simulink model "proj_pid"  (R2021a)
settings: Solver=VariableStepAuto  StartTime=0.0  StopTime=1000  RelTol=1e-3
values from neighbouring files (symbols this model uses):
  A = [0 0 1 0 ... (first row only)    [proj_LQRcode.m]    (also in proj_PIDcode.m)
  B = [0 0 ... (first row only)    [proj_LQRcode.m]    (also in proj_PIDcode.m)
  C = [1 0 0 0 ... (first row only)    [proj_LQRcode.m]    (also in proj_PIDcode.m)
  initialstate = [-3.1;-39.16;0.00002;0.0041]    [proj_PIDcode.m]
  kd1 = 500    [proj_PIDcode.m]
  kd2 = 150.643    [proj_PIDcode.m]
  ki1 = 1.7    [proj_PIDcode.m]
  ki2 = 0.005    [proj_PIDcode.m]
  kp1 = 4.5    [proj_PIDcode.m]
  kp2 = 1.35    [proj_PIDcode.m]
settings Model: Creator=huangzijing  LastModifiedBy=huangzijing

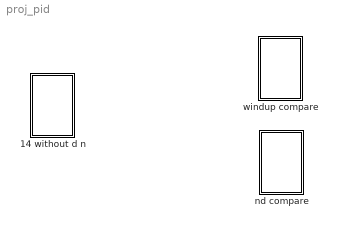
== system proj_pid ==
  14 without d n : Subsystem
  nd compare : Subsystem
  windup compare : Subsystem

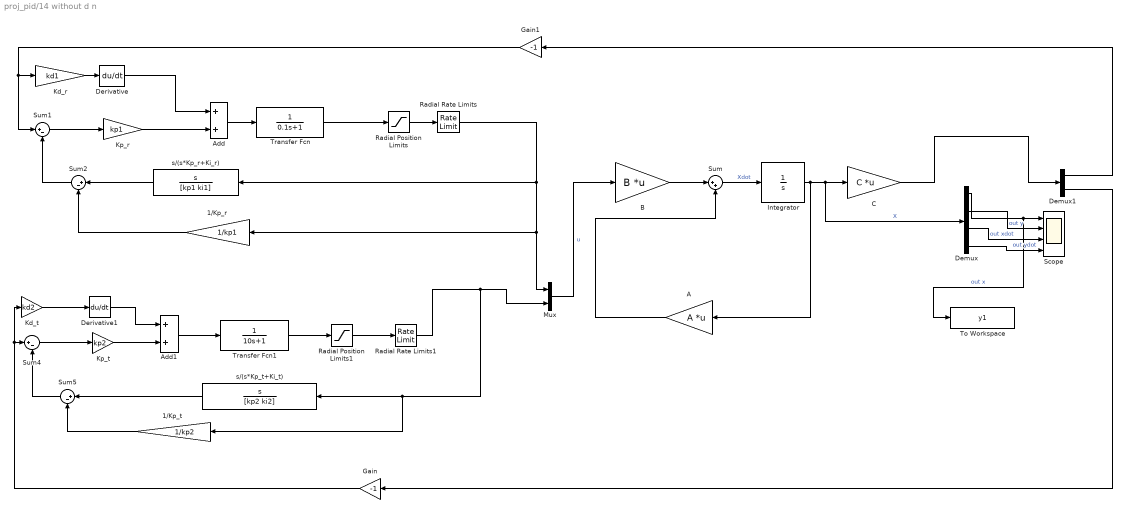
== system proj_pid/14 without d n ==
  1/Kp_r : Gain  Gain=1/kp1
  1/Kp_t : Gain  Gain=1/kp2
  A : Gain  Gain=A  Multiplication=Matrix(K*u)
  Add : Sum
  Add1 : Sum
  B : Gain  Gain=B  Multiplication=Matrix(K*u)
  C : Gain  Gain=C  Multiplication=Matrix(K*u)
  Demux : Demux
  Demux1 : Demux  Outputs=2
  Derivative : Derivative
  Derivative1 : Derivative
  Gain : Gain  Gain=-1
  Gain1 : Gain  Gain=-1
  Integrator : Integrator  InitialCondition=initialstate
  Kd_r : Gain  Gain=kd1
  Kd_t : Gain  Gain=kd2
  Kp_r : Gain  Gain=kp1
  Kp_t : Gain  Gain=kp2
  Mux : Mux  Inputs=2
  Radial Position Limits : Saturate  UpperLimit=5880  LowerLimit=-5880
  Radial Position Limits1 : Saturate  UpperLimit=820  LowerLimit=-820
  Radial Rate Limits : RateLimiter  RisingSlewLimit=30  FallingSlewLimit=-30  SampleTimeMode=inherited
  Radial Rate Limits1 : RateLimiter  RisingSlewLimit=500  FallingSlewLimit=-500  SampleTimeMode=inherited
  Scope : Scope  NumInputPorts=4
  Sum : Sum  Inputs=|++
  Sum{1..2,4..5} (4 alike) : Sum  Inputs=|+-
  To Workspace : ToWorkspace  VariableName=y1  SaveFormat=Timeseries  SampleTime=-1
  Transfer Fcn : TransferFcn  Denominator=[0.1 1]
  Transfer Fcn1 : TransferFcn  Denominator=[10 1]
  s/(s*Kp_r+Ki_r) : TransferFcn  Numerator=[1 0]  Denominator=[kp1 ki1]
  s/(s*Kp_t+Ki_t) : TransferFcn  Numerator=[1 0]  Denominator=[kp2 ki2]
  wires:
  Demux/3 -> Scope/3  "out xdot"
  Radial Position Limits1/1 -> Radial Rate Limits1/1
  Mux/1 -> B/1  "u"
  Sum/1 -> Integrator/1  "Xdot"
  Transfer Fcn1/1 -> Radial Position Limits1/1
  Add/1 -> Transfer Fcn/1
  A/1 -> Sum/2
  Derivative1/1 -> Add1/1
  s/(s*Kp_t+Ki_t)/1 -> Sum5/1
  s/(s*Kp_r+Ki_r)/1 -> Sum2/1
  1/Kp_r/1 -> Sum2/2
  Demux1/1 -> Gain1/1
  Gain/1 -> Kd_t/1, Sum4/1
  Sum2/1 -> Sum1/2
  Demux/4 -> Scope/4  "out ydot"
  Kd_t/1 -> Derivative1/1
  Add1/1 -> Transfer Fcn1/1
  Kp_t/1 -> Add1/2
  Sum1/1 -> Kp_r/1
  Sum5/1 -> Sum4/2
  B/1 -> Sum/1
  Derivative/1 -> Add/1
  Kd_r/1 -> Derivative/1
  Demux/2 -> Scope/2  "out y"
  Demux/1 -> To Workspace/1, Scope/1  "out x"
  C/1 -> Demux1/1
  Kp_r/1 -> Add/2
  Radial Position Limits/1 -> Radial Rate Limits/1
  Radial Rate Limits1/1 -> 1/Kp_t/1, s/(s*Kp_t+Ki_t)/1, Mux/2
  Integrator/1 -> Demux/1, C/1, A/1  "X"
  Gain1/1 -> Sum1/1, Kd_r/1
  Radial Rate Limits/1 -> 1/Kp_r/1, Mux/1, s/(s*Kp_r+Ki_r)/1
  Demux1/2 -> Gain/1
  1/Kp_t/1 -> Sum5/2
  Sum4/1 -> Kp_t/1
  Transfer Fcn/1 -> Radial Position Limits/1

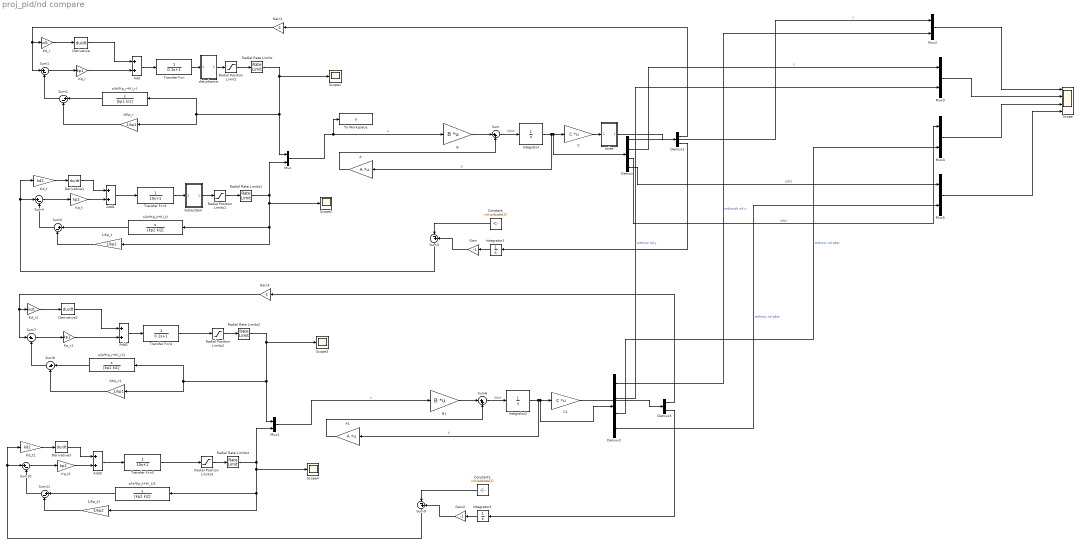
== system proj_pid/nd compare ==
  1/Kp_r : Gain  Gain=1/kp1
  1/Kp_r1 : Gain  Gain=1/kp1
  1/Kp_t : Gain  Gain=1/kp2
  1/Kp_t1 : Gain  Gain=1/kp2
  A : Gain  Gain=A  Multiplication=Matrix(K*u)
  A1 : Gain  Gain=A  Multiplication=Matrix(K*u)
  Add{,1..3} (4 alike) : Sum
  B : Gain  Gain=B  Multiplication=Matrix(K*u)
  B1 : Gain  Gain=B  Multiplication=Matrix(K*u)
  C : Gain  Gain=C  Multiplication=Matrix(K*u)
  C1 : Gain  Gain=C  Multiplication=Matrix(K*u)
  Constant : Constant  Value=initialstate(2)
  Constant1 : Constant  Value=initialstate(2)
  Demux : Demux
  Demux1 : Demux  Outputs=2
  Demux2 : Demux
  Demux3 : Demux  Outputs=2
  Derivative{,1..3} (4 alike) : Derivative
  Gain{,1..3} (4 alike) : Gain  Gain=-1
  Integrator : Integrator  InitialCondition=initialstate
  Integrator1 : Integrator
  Integrator2 : Integrator  InitialCondition=initialstate
  Integrator3 : Integrator
  Kd_r : Gain  Gain=kd1
  Kd_r1 : Gain  Gain=kd1
  Kd_t : Gain  Gain=kd2
  Kd_t1 : Gain  Gain=kd2
  Kp_r : Gain  Gain=kp1
  Kp_r1 : Gain  Gain=kp1
  Kp_t : Gain  Gain=kp2
  Kp_t1 : Gain  Gain=kp2
  Mux{,1..5} (6 alike) : Mux  Inputs=2
  Radial Position Limits : Saturate  UpperLimit=5880  LowerLimit=-5880
  Radial Position Limits1 : Saturate  UpperLimit=820  LowerLimit=-820
  Radial Position Limits2 : Saturate  UpperLimit=5880  LowerLimit=-5880
  Radial Position Limits3 : Saturate  UpperLimit=820  LowerLimit=-820
  Radial Rate Limits : RateLimiter  RisingSlewLimit=30  FallingSlewLimit=-30  SampleTimeMode=inherited
  Radial Rate Limits1 : RateLimiter  RisingSlewLimit=500  FallingSlewLimit=-500  SampleTimeMode=inherited
  Radial Rate Limits2 : RateLimiter  RisingSlewLimit=30  FallingSlewLimit=-30  SampleTimeMode=inherited
  Radial Rate Limits3 : RateLimiter  RisingSlewLimit=500  FallingSlewLimit=-500  SampleTimeMode=inherited
  Scope : Scope  NumInputPorts=4
  Scope{1..4} (4 alike) : Scope
  Subsystem : Subsystem
  Sum : Sum  Inputs=|++
  Sum{1..2,4..5,7..8,10..11} (8 alike) : Sum  Inputs=|+-
  Sum3 : Sum  Inputs=|-+
  Sum6 : Sum  Inputs=|++
  Sum9 : Sum  Inputs=|-+
  To Workspace : ToWorkspace  VariableName=u  SampleTime=-1
      settings: Save2DSignal=2-D array (concatenate along first dimension)
  Transfer Fcn : TransferFcn  Denominator=[0.1 1]
  Transfer Fcn1 : TransferFcn  Denominator=[10 1]
  Transfer Fcn2 : TransferFcn  Denominator=[0.1 1]
  Transfer Fcn3 : TransferFcn  Denominator=[10 1]
  disturbance : Subsystem
  "noise " : Subsystem
  s/(s*Kp_r+Ki_r) : TransferFcn  Numerator=[1 0]  Denominator=[kp1 ki1]
  s/(s*Kp_r+Ki_r)1 : TransferFcn  Numerator=[1 0]  Denominator=[kp1 ki1]
  s/(s*Kp_t+Ki_t) : TransferFcn  Numerator=[1 0]  Denominator=[kp2 ki2]
  s/(s*Kp_t+Ki_t)1 : TransferFcn  Numerator=[1 0]  Denominator=[kp2 ki2]
  wires:
  Sum6/1 -> Integrator2/1  "Xdot"
  Integrator3/1 -> Gain2/1
  Demux2/4 -> Mux5/2  "without nd ydot"
  Sum2/1 -> Sum1/2
  Demux1/1 -> Gain1/1
  Sum11/1 -> Sum10/2
  B1/1 -> Sum6/1
  Demux3/1 -> Gain3/1
  Radial Position Limits2/1 -> Radial Rate Limits2/1
  Sum4/1 -> Kp_t/1
  Transfer Fcn2/1 -> Radial Position Limits2/1
  Mux/1 -> To Workspace/1, B/1  "u"
  Add/1 -> Transfer Fcn/1
  Demux2/1 -> Mux2/2  "withouth nd x"
  s/(s*Kp_t+Ki_t)1/1 -> Sum11/1
  Integrator/1 -> Demux/1, C/1, A/1  "X"
  Transfer Fcn3/1 -> Radial Position Limits3/1
  Constant/1 -> Sum3/1
  Transfer Fcn1/1 -> Subsystem/1(In1)
  Kd_r1/1 -> Derivative2/1
  Radial Position Limits/1 -> Radial Rate Limits/1
  Derivative3/1 -> Add3/1
  Mux3/1 -> Scope/2
  Transfer Fcn/1 -> disturbance/1(In1)
  Add3/1 -> Transfer Fcn3/1
  Mux1/1 -> B1/1  "u"
  Demux2/3 -> Mux4/2  "without nd xdot"
  s/(s*Kp_r+Ki_r)1/1 -> Sum8/1
  Sum10/1 -> Kp_t1/1
  1/Kp_t/1 -> Sum5/2
  Sum1/1 -> Kp_r/1
  1/Kp_r1/1 -> Sum8/2
  Kp_t1/1 -> Add3/2
  Mux4/1 -> Scope/3
  s/(s*Kp_r+Ki_r)/1 -> Sum2/1
  Gain1/1 -> Sum1/1, Kd_r/1
  Demux/4 -> Mux5/1  "ydot"
  Gain2/1 -> Sum9/2
  Kp_t/1 -> Add1/2
  Derivative1/1 -> Add1/1
  1/Kp_t1/1 -> Sum11/2
  Sum/1 -> Integrator/1  "Xdot"
  Sum8/1 -> Sum7/2
  Sum3/1 -> Kd_t/1, Sum4/1
  Gain3/1 -> Sum7/1, Kd_r1/1
  Sum5/1 -> Sum4/2
  Constant1/1 -> Sum9/1
  1/Kp_r/1 -> Sum2/2
  Radial Position Limits3/1 -> Radial Rate Limits3/1
  Mux5/1 -> Scope/4
  Radial Rate Limits3/1 -> Scope4/1, s/(s*Kp_t+Ki_t)1/1, 1/Kp_t1/1, Mux1/2
  Sum9/1 -> Kd_t1/1, Sum10/1
  B/1 -> Sum/1
  Kp_r/1 -> Add/2
  Derivative/1 -> Add/1
  Demux/3 -> Mux4/1  "xdot"
  Subsystem/1(Out1) -> Radial Position Limits1/1
  C/1 -> "noise "/1(In1)
  Radial Rate Limits1/1 -> Scope2/1, s/(s*Kp_t+Ki_t)/1, 1/Kp_t/1, Mux/2
  "noise "/1(Out1) -> Demux1/1
  Demux/2 -> Mux3/1  "y"
  A/1 -> Sum/2
  Kd_t1/1 -> Derivative3/1
  Demux/1 -> Mux2/1  "x"
  Demux1/2 -> Integrator1/1
  Radial Rate Limits2/1 -> Scope3/1, s/(s*Kp_r+Ki_r)1/1, 1/Kp_r1/1, Mux1/1
  Mux2/1 -> Scope/1
  Add2/1 -> Transfer Fcn2/1
  Gain/1 -> Sum3/2
  Add1/1 -> Transfer Fcn1/1
  s/(s*Kp_t+Ki_t)/1 -> Sum5/1
  Kd_r/1 -> Derivative/1
  Demux2/2 -> Mux3/2  "without nd y"
  C1/1 -> Demux3/1
  Derivative2/1 -> Add2/1
  Radial Position Limits1/1 -> Radial Rate Limits1/1
  Kd_t/1 -> Derivative1/1
  Radial Rate Limits/1 -> Scope1/1, s/(s*Kp_r+Ki_r)/1, 1/Kp_r/1, Mux/1
  Integrator2/1 -> Demux2/1, C1/1, A1/1  "X"
  Demux3/2 -> Integrator3/1
  Kp_r1/1 -> Add2/2
  Sum7/1 -> Kp_r1/1
  disturbance/1(Out1) -> Radial Position Limits/1
  A1/1 -> Sum6/2
  Integrator1/1 -> Gain/1

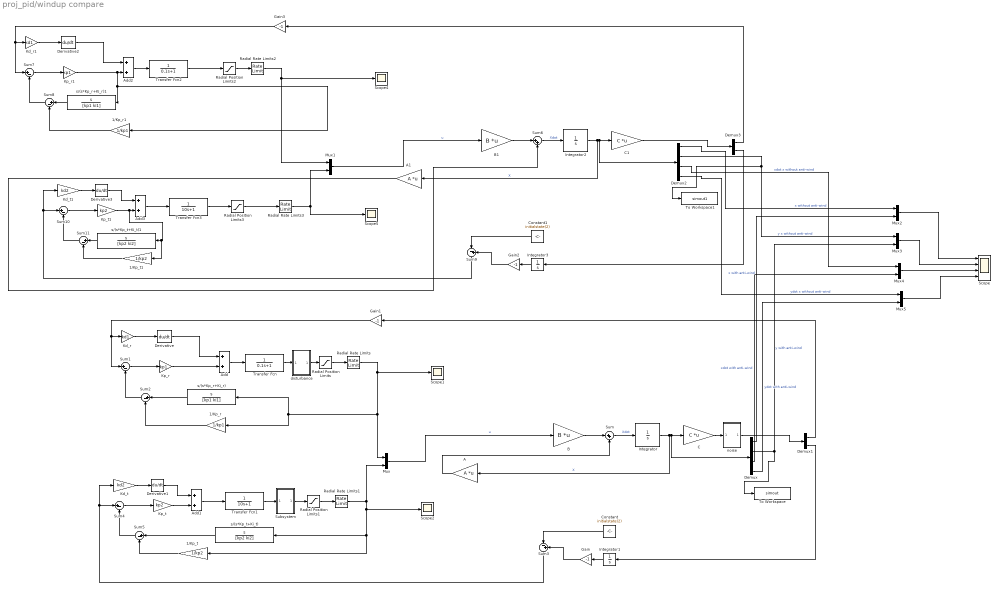
== system proj_pid/windup compare ==
  1/Kp_r : Gain  Gain=1/kp1
  1/Kp_r1 : Gain  Gain=1/kp1
  1/Kp_t : Gain  Gain=1/kp2
  1/Kp_t1 : Gain  Gain=1/kp2
  A : Gain  Gain=A  Multiplication=Matrix(K*u)
  A1 : Gain  Gain=A  Multiplication=Matrix(K*u)
  Add{,1..3} (4 alike) : Sum
  B : Gain  Gain=B  Multiplication=Matrix(K*u)
  B1 : Gain  Gain=B  Multiplication=Matrix(K*u)
  C : Gain  Gain=C  Multiplication=Matrix(K*u)
  C1 : Gain  Gain=C  Multiplication=Matrix(K*u)
  Constant : Constant  Value=initialstate(2)
  Constant1 : Constant  Value=initialstate(2)
  Demux : Demux
  Demux1 : Demux  Outputs=2
  Demux2 : Demux
  Demux3 : Demux  Outputs=2
  Derivative{,1..3} (4 alike) : Derivative
  Gain{,1..3} (4 alike) : Gain  Gain=-1
  Integrator : Integrator  InitialCondition=initialstate
  Integrator1 : Integrator
  Integrator2 : Integrator  InitialCondition=initialstate
  Integrator3 : Integrator
  Kd_r : Gain  Gain=kd1
  Kd_r1 : Gain  Gain=kd1
  Kd_t : Gain  Gain=kd2
  Kd_t1 : Gain  Gain=kd2
  Kp_r : Gain  Gain=kp1
  Kp_r1 : Gain  Gain=kp1
  Kp_t : Gain  Gain=kp2
  Kp_t1 : Gain  Gain=kp2
  Mux{,1..5} (6 alike) : Mux  Inputs=2
  Radial Position Limits : Saturate  UpperLimit=5880  LowerLimit=-5880
  Radial Position Limits1 : Saturate  UpperLimit=820  LowerLimit=-820
  Radial Position Limits2 : Saturate  UpperLimit=5880  LowerLimit=-5880
  Radial Position Limits3 : Saturate  UpperLimit=820  LowerLimit=-820
  Radial Rate Limits : RateLimiter  RisingSlewLimit=30  FallingSlewLimit=-30  SampleTimeMode=inherited
  Radial Rate Limits1 : RateLimiter  RisingSlewLimit=500  FallingSlewLimit=-500  SampleTimeMode=inherited
  Radial Rate Limits2 : RateLimiter  RisingSlewLimit=30  FallingSlewLimit=-30  SampleTimeMode=inherited
  Radial Rate Limits3 : RateLimiter  RisingSlewLimit=500  FallingSlewLimit=-500  SampleTimeMode=inherited
  Scope : Scope  NumInputPorts=4
  Scope{1..2,4..5} (4 alike) : Scope
  Subsystem : Subsystem
  Sum : Sum  Inputs=|++
  Sum{1..2,4..5,7..8,10..11} (8 alike) : Sum  Inputs=|+-
  Sum3 : Sum  Inputs=|-+
  Sum6 : Sum  Inputs=|++
  Sum9 : Sum  Inputs=|-+
  To Workspace : ToWorkspace  VariableName=simout  SaveFormat=Timeseries  SampleTime=-1
  To Workspace1 : ToWorkspace  VariableName=simout1  SaveFormat=Timeseries  SampleTime=-1
  Transfer Fcn : TransferFcn  Denominator=[0.1 1]
  Transfer Fcn1 : TransferFcn  Denominator=[10 1]
  Transfer Fcn2 : TransferFcn  Denominator=[0.1 1]
  Transfer Fcn3 : TransferFcn  Denominator=[10 1]
  disturbance : Subsystem
  "noise " : Subsystem
  s/(s*Kp_r+Ki_r) : TransferFcn  Numerator=[1 0]  Denominator=[kp1 ki1]
  s/(s*Kp_r+Ki_r)1 : TransferFcn  Numerator=[1 0]  Denominator=[kp1 ki1]
  s/(s*Kp_t+Ki_t) : TransferFcn  Numerator=[1 0]  Denominator=[kp2 ki2]
  s/(s*Kp_t+Ki_t)1 : TransferFcn  Numerator=[1 0]  Denominator=[kp2 ki2]
  wires:
  Sum/1 -> Integrator/1  "Xdot"
  B/1 -> Sum/1
  Integrator/1 -> Demux/1, C/1, A/1  "X"
  A/1 -> Sum/2
  Radial Rate Limits/1 -> Scope1/1, s/(s*Kp_r+Ki_r)/1, 1/Kp_r/1, Mux/1
  1/Kp_r/1 -> Sum2/2
  Kp_t/1 -> Add1/2
  Radial Position Limits/1 -> Radial Rate Limits/1
  Radial Position Limits1/1 -> Radial Rate Limits1/1
  Sum5/1 -> Sum4/2
  Radial Rate Limits1/1 -> Scope2/1, s/(s*Kp_t+Ki_t)/1, 1/Kp_t/1, Mux/2
  Sum2/1 -> Sum1/2
  1/Kp_t/1 -> Sum5/2
  Add/1 -> Transfer Fcn/1
  s/(s*Kp_r+Ki_r)/1 -> Sum2/1
  Kp_r/1 -> Add/2
  Derivative1/1 -> Add1/1
  Sum4/1 -> Kp_t/1
  Sum1/1 -> Kp_r/1
  Kd_t/1 -> Derivative1/1
  Kd_r/1 -> Derivative/1
  Add1/1 -> Transfer Fcn1/1
  s/(s*Kp_t+Ki_t)/1 -> Sum5/1
  Derivative/1 -> Add/1
  Mux/1 -> B/1  "u"
  Sum3/1 -> Kd_t/1, Sum4/1
  Demux1/2 -> Integrator1/1
  Constant/1 -> Sum3/1
  Integrator1/1 -> Gain/1
  Gain/1 -> Sum3/2
  Demux/2 -> Mux3/2, To Workspace/1  "y with anti-wind"
  Demux1/1 -> Gain1/1
  Gain1/1 -> Sum1/1, Kd_r/1
  Integrator3/1 -> Gain2/1
  Sum7/1 -> Kp_r1/1
  Kd_r1/1 -> Derivative2/1
  Integrator2/1 -> Demux2/1, C1/1, A1/1  "X"
  B1/1 -> Sum6/1
  Gain2/1 -> Sum9/2
  Sum6/1 -> Integrator2/1  "Xdot"
  Sum10/1 -> Kp_t1/1
  Radial Rate Limits2/1 -> Scope4/1, Mux1/1
  Radial Position Limits2/1 -> Radial Rate Limits2/1
  Mux1/1 -> B1/1  "u"
  Kp_t1/1 -> 1/Kp_t1/1, s/(s*Kp_t+Ki_t)1/1, Add3/2
  1/Kp_r1/1 -> Sum8/2
  Sum11/1 -> Sum10/2
  Radial Position Limits3/1 -> Radial Rate Limits3/1
  Radial Rate Limits3/1 -> Scope5/1, Mux1/2
  Sum8/1 -> Sum7/2
  Demux3/2 -> Integrator3/1
  1/Kp_t1/1 -> Sum11/2
  Demux2/1 -> Mux2/1  "x without anti-wind"
  Derivative3/1 -> Add3/1
  C1/1 -> Demux3/1
  Transfer Fcn3/1 -> Radial Position Limits3/1
  Kd_t1/1 -> Derivative3/1
  Add3/1 -> Transfer Fcn3/1
  s/(s*Kp_t+Ki_t)1/1 -> Sum11/1
  Transfer Fcn2/1 -> Radial Position Limits2/1
  Demux2/4 -> Mux5/1  "ydot x without anti-wind"
  Sum9/1 -> Kd_t1/1, Sum10/1
  Constant1/1 -> Sum9/1
  Kp_r1/1 -> 1/Kp_r1/1, s/(s*Kp_r+Ki_r)1/1, Add2/2
  A1/1 -> Sum6/2
  Demux2/2 -> Mux3/1, To Workspace1/1  "y x without anti-wind"
  Add2/1 -> Transfer Fcn2/1
  s/(s*Kp_r+Ki_r)1/1 -> Sum8/1
  Demux2/3 -> Mux4/1  "xdot x without anti-wind"
  Demux3/1 -> Gain3/1
  Gain3/1 -> Sum7/1, Kd_r1/1
  Derivative2/1 -> Add2/1
  Demux/1 -> Mux2/2  "x with anti-wind"
  Demux/3 -> Mux4/2  "xdot with anti-wind"
  Demux/4 -> Mux5/2  "ydot with anti-wind"
  Mux2/1 -> Scope/1
  Mux3/1 -> Scope/2
  Mux4/1 -> Scope/3
  Mux5/1 -> Scope/4
  Transfer Fcn/1 -> disturbance/1(In1)
  disturbance/1(Out1) -> Radial Position Limits/1
  Transfer Fcn1/1 -> Subsystem/1(In1)
  Subsystem/1(Out1) -> Radial Position Limits1/1
  C/1 -> "noise "/1(In1)
  "noise "/1(Out1) -> Demux1/1

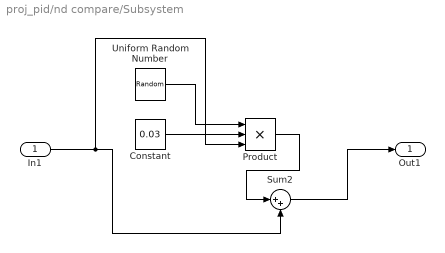
== system proj_pid/nd compare/Subsystem ==
  In1 : Inport
  Constant : Constant  Value=0.03
  Product : Product  Inputs=3
  Sum2 : Sum  Inputs=|++
  Uniform Random Number : UniformRandomNumber  SampleTime=0.1
  Out1 : Outport
  wires:
  Sum2/1 -> Out1/1
  Constant/1 -> Product/2
  Uniform Random Number/1 -> Product/1
  In1/1 -> Sum2/2, Product/3
  Product/1 -> Sum2/1

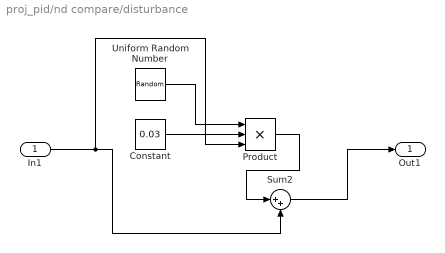
== system proj_pid/nd compare/disturbance ==
  In1 : Inport
  Constant : Constant  Value=0.03
  Product : Product  Inputs=3
  Sum2 : Sum  Inputs=|++
  Uniform Random Number : UniformRandomNumber  SampleTime=0.1
  Out1 : Outport
  wires:
  Sum2/1 -> Out1/1
  Constant/1 -> Product/2
  Uniform Random Number/1 -> Product/1
  In1/1 -> Sum2/2, Product/3
  Product/1 -> Sum2/1

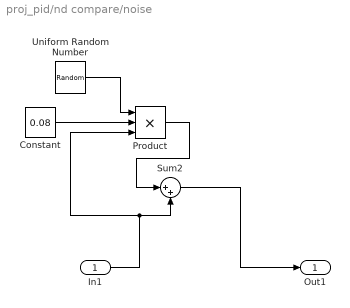
== system proj_pid/nd compare/noise  ==
  In1 : Inport
  Constant : Constant  Value=0.08
  Product : Product  Inputs=3
  Sum2 : Sum  Inputs=|++
  Uniform Random Number : UniformRandomNumber  SampleTime=0.1
  Out1 : Outport
  wires:
  Constant/1 -> Product/2
  Uniform Random Number/1 -> Product/1
  Sum2/1 -> Out1/1
  In1/1 -> Sum2/2, Product/3
  Product/1 -> Sum2/1

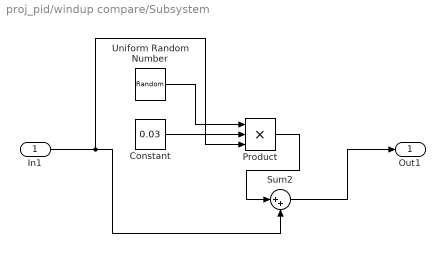
== system proj_pid/windup compare/Subsystem ==
  In1 : Inport
  Constant : Constant  Value=0.03
  Product : Product  Inputs=3
  Sum2 : Sum  Inputs=|++
  Uniform Random Number : UniformRandomNumber  SampleTime=0.1
  Out1 : Outport
  wires:
  Sum2/1 -> Out1/1
  Constant/1 -> Product/2
  Uniform Random Number/1 -> Product/1
  In1/1 -> Sum2/2, Product/3
  Product/1 -> Sum2/1

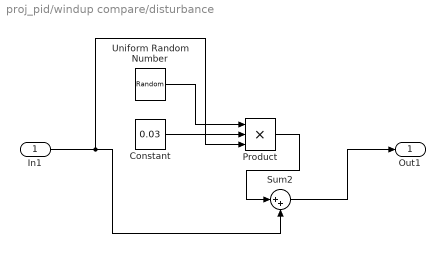
== system proj_pid/windup compare/disturbance ==
  In1 : Inport
  Constant : Constant  Value=0.03
  Product : Product  Inputs=3
  Sum2 : Sum  Inputs=|++
  Uniform Random Number : UniformRandomNumber  SampleTime=0.1
  Out1 : Outport
  wires:
  Sum2/1 -> Out1/1
  Constant/1 -> Product/2
  Uniform Random Number/1 -> Product/1
  In1/1 -> Sum2/2, Product/3
  Product/1 -> Sum2/1

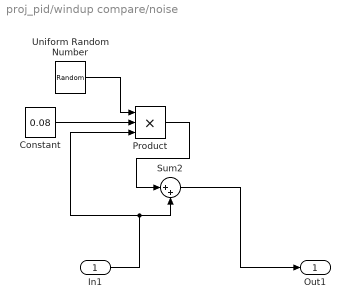
== system proj_pid/windup compare/noise  ==
  In1 : Inport
  Constant : Constant  Value=0.08
  Product : Product  Inputs=3
  Sum2 : Sum  Inputs=|++
  Uniform Random Number : UniformRandomNumber  SampleTime=0.1
  Out1 : Outport
  wires:
  Constant/1 -> Product/2
  Uniform Random Number/1 -> Product/1
  Sum2/1 -> Out1/1
  In1/1 -> Sum2/2, Product/3
  Product/1 -> Sum2/1
